simulink model "broken_tooth_gear"  (R2019b)
settings: Solver=VariableStepAuto  StartTime=0.0  StopTime=10  RelTol=1e-3
undefined symbols (not defined in the file or in its folder): sigbuilder_block
settings Model: Creator=User  LastModifiedBy=User

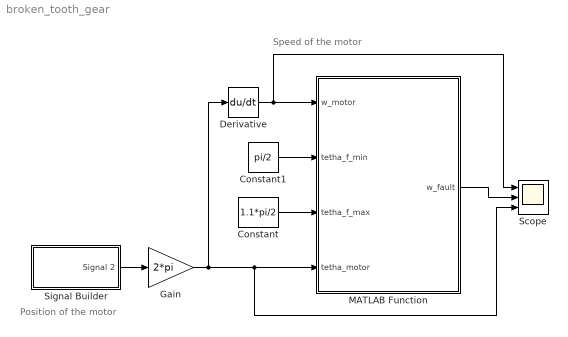
== system broken_tooth_gear ==
  note: Speed of the motor
  note: Position of the motor
  Constant : Constant  Value=1.1*pi/2
  Constant1 : Constant  Value=pi/2
  Derivative : Derivative
  Gain : Gain  Gain=2*pi
  MATLAB Function : MATLAB Function  TreatAsAtomicUnit=on
  Scope : Scope  NumInputPorts=3
  Signal Builder : Subsystem  Tag=STV Subsys  LoadFcn=sigbuilder_block('load');  StartFcn=sigbuilder_block('start');  StopFcn=sigbuilder_block('stop');  ClipboardFcn=sigbuilder_block('clipboard');  mask(Sigbuilder block){tuvar=[0:10]}
      mask help: Simulink:masks:SigbuilderBlock_MD
      mask init:
      | if ~strcmp(get_param(bdroot(gcbh),'SimulationStatus'),'stopped') tuvar = sigbuilder_block('maskInit'); end
      settings: CopyFcn=sigbuilder_block('copy');  DeleteFcn=sigbuilder_block('delete');  ModelCloseFcn=sigbuilder_block('modelClose');  PreSaveFcn=sigbuilder_block('preSave');  PauseFcn=sigbuilder_block('pause');  ContinueFcn=sigbuilder_block('continue');  NameChangeFcn=sigbuilder_block('namechange');  OpenFcn=sigbuilder_block('open',[437.6 199.2 550.4 400 ]);  CloseFcn=sigbuilder_block('close');
      mask Display: plot(0, 0, 100, 100,[2, 2, 32, 32, 2], [68, 8, 8, 68, 68],[32, 2], [38, 38], [32, 19, 2],[53, 60, 44], [32, 17, 17, 2],[16, 16, 31, 31]);txt = getActiveGroup(gcbh);text(2, 100, txt,'verticalAlignment', 'top');
  wires:
  Constant1/1 -> MATLAB Function/2(tetha_f_min)
  Constant/1 -> MATLAB Function/3(tetha_f_max)
  MATLAB Function/1(w_fault) -> Scope/2
  Gain/1 -> Scope/3, MATLAB Function/4(tetha_motor), Derivative/1
  Derivative/1 -> Scope/1, MATLAB Function/1(w_motor)
  Signal Builder/1(Signal 2) -> Gain/1

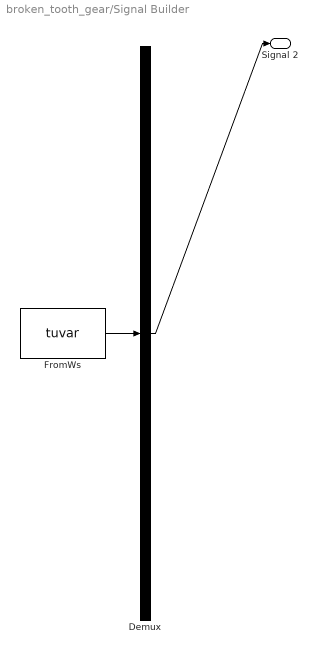
== system broken_tooth_gear/Signal Builder ==
  Demux : Demux  Tag=STV Demux  Outputs=1
  FromWs : FromWorkspace  Tag=STV FromWs  VariableName=tuvar  SampleTime=0
      SigBuilderData=|
      | common.afterFinalStr = 'Extrapolate'
      | common.sampleTime = 0
      | dataSet.timeRange = [0 10]
      | dataSet.name = 'Group 1'
      | sbobj.Groups.Name = 'Group 1'
      | sbobj.Groups.Signals.Name = 'Signal 2'
      | sbobj.Groups.Signals.XData = [0 1 2 4 6 8 10]
      | sbobj.Groups.Signals.YData = [0 0.025 0.06 0.165 0.3 0.595 1]
  Signal 2 : Outport  Tag=STV Outport
  wires:
  FromWs/1 -> Demux/1
  Demux/1 -> Signal 2/1

== matlab function broken_tooth_gear/MATLAB Function ==
  data: w_motor input; w_fault output; tetha_f_min input; tetha_f_max input; tetha_motor input
function w_fault = Broken_Tooth(w_motor,tetha_f_min,tetha_f_max,tetha_motor)

w_fault=0;


if ((tetha_motor*360/(2*pi)) > (tetha_f_min*360/(2*pi)))&((tetha_motor*360/(2*pi)) < (tetha_f_max*360/(2*pi)))
    
    for c=1:((tetha_f_max*360/(2*pi))-(tetha_f_min*360/(2*pi)))
        
        w_motor = w_motor + (w_motor/314)*((tetha_f_max*360/(2*pi))-(tetha_f_min*360/(2*pi)));
        w_fault = w_motor;
            
    end
    
else 
    w_fault = w_motor;
end
